simulink model "calc_diff"  (R2021a)
settings: Solver=VariableStepAuto  StartTime=0.0  StopTime=10.0  RelTol=1e-3
values from neighbouring files (symbols this model uses):
  s_type = 3    [script_main.m]
  Ts = 1e-2    (= 0.01)    [script_main.m]    (also in skryptv1.m; skryptv2.m)
undefined symbols (not defined in the file or in its folder): sigbuilder_block
libraries: cstblocks x2
settings Model: Creator=mokro  LastModifiedBy=mokro

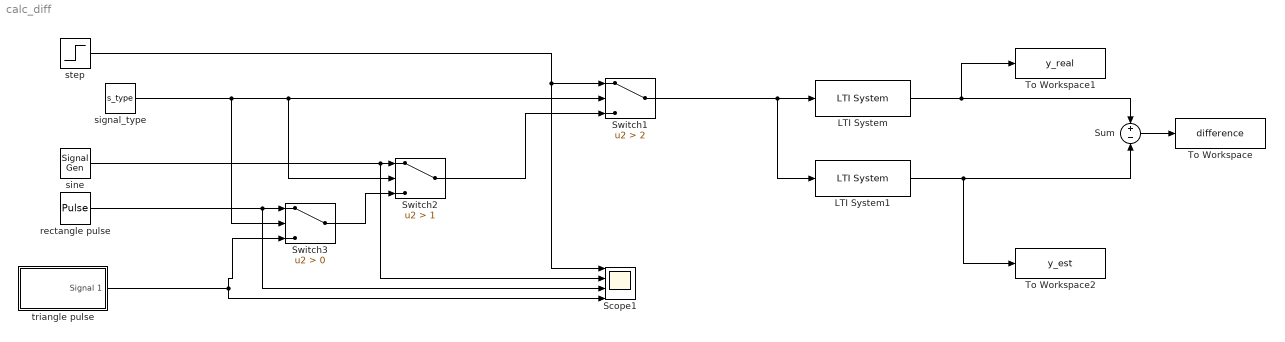
== system calc_diff ==
  LTI System : cstblocks/LTI System  sys=Gd  IC=[]
  LTI System1 : cstblocks/LTI System  sys=Gdf  IC=[]
  Scope1 : Scope  NumInputPorts=4
  Sum : Sum  Inputs=+-
  Switch1 : Switch  Criteria=u2 > Threshold  Threshold=2
  Switch2 : Switch  Criteria=u2 > Threshold  Threshold=1
  Switch3 : Switch  Criteria=u2 > Threshold
  To Workspace : ToWorkspace  VariableName=difference  SaveFormat=Timeseries  SampleTime=Ts
  To Workspace1 : ToWorkspace  VariableName=y_real  SaveFormat=Timeseries  SampleTime=Ts
  To Workspace2 : ToWorkspace  VariableName=y_est  SaveFormat=Timeseries  SampleTime=Ts
  rectangle pulse : DiscretePulseGenerator  PulseType=Time based  Period=10  PulseWidth=10  PhaseDelay=1
  signal_type : Constant  Value=s_type
  sine : SignalGenerator  Frequency=2  Units=rad/sec
  step : Step  SampleTime=0
  triangle pulse : Subsystem  Tag=STV Subsys  LoadFcn=sigbuilder_block('load');  StartFcn=sigbuilder_block('start');  StopFcn=sigbuilder_block('stop');  ClipboardFcn=sigbuilder_block('clipboard');  mask(Sigbuilder block){tuvar=[0:10]}
      mask help: Simulink:masks:SigbuilderBlock_MD
      mask init:
      | if ~strcmp(get_param(bdroot(gcbh),'SimulationStatus'),'stopped') tuvar = sigbuilder_block('maskInit'); end
      settings: CopyFcn=sigbuilder_block('copy');  DeleteFcn=sigbuilder_block('delete');  ModelCloseFcn=sigbuilder_block('modelClose');  PreSaveFcn=sigbuilder_block('preSave');  PauseFcn=sigbuilder_block('pause');  ContinueFcn=sigbuilder_block('continue');  NameChangeFcn=sigbuilder_block('namechange');  OpenFcn=sigbuilder_block('open',[437.6 199.2 550.4 400 ]);  CloseFcn=sigbuilder_block('close');
      mask Display: plot(0, 0, 100, 100,[2, 2, 32, 32, 2], [68, 8, 8, 68, 68],[32, 2], [38, 38], [32, 19, 2],[53, 60, 44], [32, 17, 17, 2],[16, 16, 31, 31]);txt = getActiveGroup(gcbh);text(2, 100, txt,'verticalAlignment', 'top');
  wires:
  LTI System/1 -> To Workspace1/1, Sum/1
  LTI System1/1 -> To Workspace2/1, Sum/2
  Switch1/1 -> LTI System/1, LTI System1/1
  Sum/1 -> To Workspace/1
  Switch2/1 -> Switch1/3
  rectangle pulse/1 -> Scope1/3, Switch3/1
  step/1 -> Scope1/1, Switch1/1
  sine/1 -> Scope1/2, Switch2/1
  triangle pulse/1(Signal 1) -> Switch3/3, Scope1/4
  signal_type/1 -> Switch3/2, Switch2/2, Switch1/2
  Switch3/1 -> Switch2/3

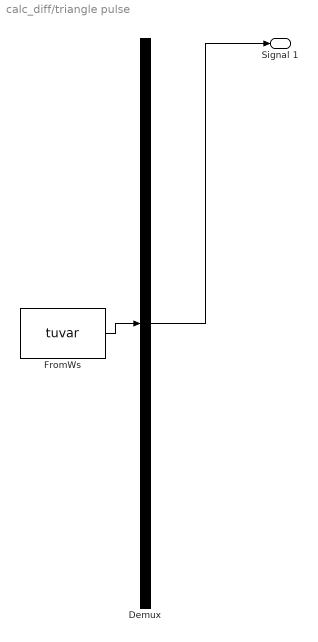
== system calc_diff/triangle pulse ==
  Demux : Demux  Tag=STV Demux  Outputs=1
      settings: DisplayOption=none
  FromWs : FromWorkspace  Tag=STV FromWs  VariableName=tuvar
      SigBuilderData=|
      | common.afterFinalStr = 'Extrapolate'
      | common.sampleTime = 0
      | dataSet.timeRange = [0 10]
      | dataSet.name = 'Group 1'
      | sbobj.Groups.Name = 'Group 1'
      | sbobj.Groups.Signals.Name = 'Signal 1'
      | sbobj.Groups.Signals.XData = [0 1 1.5 2 10]
      | sbobj.Groups.Signals.YData = [0 0 1 0 0]
  Signal 1 : Outport  Tag=STV Outport
  wires:
  Demux/1 -> Signal 1/1
  FromWs/1 -> Demux/1
